simulink model "networkAnalyzer"  (R2023a)
settings: Solver=VariableStepAuto  StartTime=0.0  StopTime=10e-6  RelTol=1e-3
StopFcn:
  | a = smith(SParamObjOut,1,1);
  | a.LineWidth = 3;
  | a.Color = 'red';
undefined symbols (not defined in the file or in its folder): S
libraries: simrfV2elements x4, simrfV2util1 x1, simrfV2testbenches x1
settings Model: Creator=Hossein  LastModifiedBy=Hossein

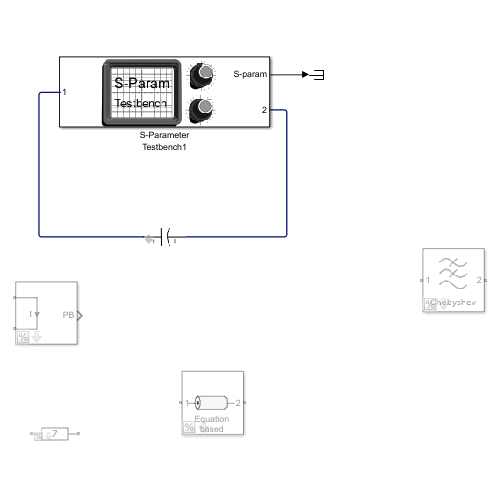
[thumbnail: Simulink's stored preview of the top-level diagram]
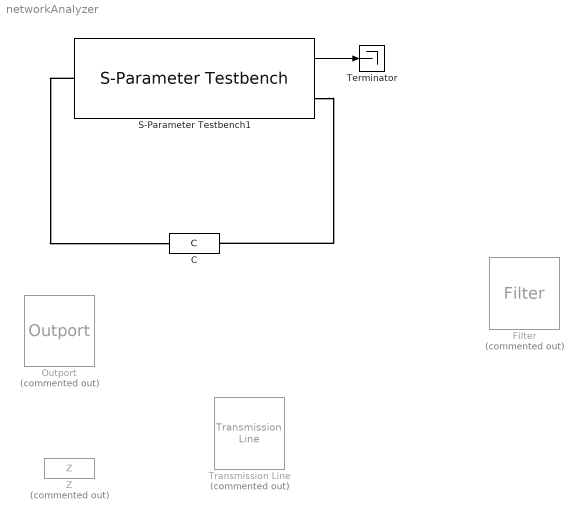
== system networkAnalyzer ==
  C : simrfV2elements/C  classname=capacitor  Capacitance=1e-12 F
  Filter : simrfV2elements/Filter  Commented=on  classname=filter  DesignMethod=Chebyshev  ResponseType=Lowpass  Implementation=LC Tee  ImplementationIdeal=Frequency domain  ImplementationRational=Transfer function  UseFilterOrder=on  FilterOrder=9  PassFreq_lp=1 GHz  PassFreq_hp=2 GHz  PassFreq_bp=[2 3] GHz  PassFreq_bs=[1 4] GHz  PassAtten=10*log10(2)  StopFreq_lp=2 GHz  StopFreq_hp=1 GHz  StopFreq_bp=[1.5 3.5] GHz  StopFreq_bs=[2.1 2.9] GHz  StopAtten=40  Rsrc=50  Rload=50  AutoImpulseLength=off  ImpulseLength=2.5e-10*2048 s  InternalGrounding=on  PlotFuncLeft=Voltage transfer  PlotLeftForm=Magnitude (dB)  PlotRightOnVT=None  PlotRightNoTD=None  PlotRightNoGD=None  PlotRightNoIR=None  PlotRightNoSR=None  PlotRightForm=Imaginary  FreqPoints=[0.75:0.005:1.25]  Freq_unit=GHz  TimePoints=linspace(0,1,1e6+1)  Time_unit=s  XaxisScale=Linear  YaxisScale=Linear  needRedraw=0
  Outport : simrfV2util1/Outport  Commented=on  SensorType=Ideal current  OutputFormat=Real Passband  CarrierFreq=0 Hz  ZL=0  InternalGrounding=off  StepSize=1e-6 s  AutoStep=on  HalfPolyphaseLength=12
  S-Parameter Testbench1 : simrfV2testbenches/S-Parameter Testbench  classname=tbsparam  UseIntConf=on  SimNoise=off  T_amp_dBm=57.0  NumOfPorts=2  MeasureAll=on  SaveS2P=0  ResetableRand=3.8155845709300840e-01  SParamElem=[2 1]  SParamElemPrev=[1 1;2 1;1 2;2 2]  SParamElem1Sel=[1 2;1 2]  SParamElem1SelMapped=[1 2;1 2]  SParamElem1Ind=[1 2 3 4]  SParamElem2Val=[1;2]  InputIdx=1  VarName=SParamObjOut  Fin=2.4e9  Base_bw=800e6  Z0=50  ShowSParam=on  ShowSParamType=Magnitude  MagSparamUnits=Auto  ReImSparamUnits=Auto  InternalGrounding=on  fft_size=1024  Nbins=128  Intermission=3  OS=8  resp=[6.81051648626987e-09;5.8024140195314e-09;3.58265522804047e-09;6.66452894173414e-10;-2.29830488147897e-09;-4.67428137407126e-09;-5.97102098277499e-09;-5.94537038448462e-09;-4.64561861711604e-09;-2.39171175919761e-09;3.02146614802531e-10;2.84404735119469e-09;4.69381960740718e-09;5.47719153734007e-09;5.06068154612974e-09;3.57243094958534e-09;1.366259939602e-09;-1.06150826708262e-09;-3.18309040418601e-09;-4.55343931798306e-09;-4.90300228845816e-09;-4.18984051338105e-09;-2.60123212249622e-09;-5.05981910450121e-10;1.63100066503767e-09;3.35323703526402e-09;4.31630712508652e-09;4.37755410273664e-09;3.67920163757939e-09;2.77705269652491e-09;2.96129531464871e-09;7.1120200677028e-09;2.18299606421558e-08;6.23598544160819e-08;1.63269316723402e-07;4.00396054651843e-07;9.33827347722446e-07;2.08835238509805e-06;4.4976610306672e-06;9.35203499698743e-06;1.8806203403848e-05;3.66229703357968e-05;6.91457717160638e-05;0.000126703493452547;0.000225544772074564;0.000390365110838636;0.000657415791880327;0.00107805759777328;0.00172243928642742;0.00268274593480174;0.00407519716603967;0.00603972153584085;0.00873605359041221;0.0123349736476851;0.0170036224447493;0.0228843469976878;0.0300674092363405;0.0385590946804533;0.0482481936534249;0.0588753004685631;0.07001061092895;0.0810465648285553;0.0912114449704557;0.0996086432816028;0.105283621788724;0.107316735371352;0.104935413468097;0.0976343544391195;0.0852882136126929;0.0682387012558636;0.0473379128100542;0.0239326874790702;-0.000219018604988352;-0.0230997807439736;-0.0426416910645372;-0.056971112585493;-0.0646584952534719;-0.0649370802195157;-0.0578540941489043;-0.0443239056926063;-0.0260644349622775;-0.00541460497265073;0.0149505083913944;0.0323719850072223;0.0445777836518677;0.0500155756815352;0.0480930698267642;0.0392823992156686;0.0250646998199902;0.00771614495830684;-0.0100366513630653;-0.0254404652060814;-0.0361512573431075;-0.040609750820403;-0.0382921967767228;-0.0297911168058924;-0.0167090442506466;-0.00138061048714176;0.0135310307206473;0.0254941930020491;0.0325445139287934;0.0336192652264231;0.0287301008754187;0.0189429989120413;0.00616915572758517;-0.00719464495852944;-0.0187097218303718;-0.026341060203831;-0.0288222277716438;-0.0258723892394917;-0.0182262540822959;-0.00747337715649778;0.00426051684671593;0.0147276156491389;0.0219872110759769;0.0247675993169048;0.0226921959767603;0.016328516091456;0.00705365723689313;-0.00323418431282428;-0.0124989378643042;-0.0189677294627156;-0.0214706685012344;-0.0196536986000975;-0.0140251942169414;-0.00583074630236407;0.00321509414775467;0.0112833612309266;0.016798652509765;0.018746530708132;0.0168601233351881;0.011651374043514;0.00428455388818464;-0.00367838381766407;-0.0106057322490685;-0.0151287962375505;-0.0164117263387738;-0.0143051567759723;-0.00935544535559019;-0.00267156669410891;0.00431917801823937;0.0101734666305566;0.0137285836066262;0.0143325356565713;0.0119621592417434;0.00720806812700198;0.00113337976038217;-0.00496091995827656;-0.00981268853205416;-0.0124588389122865;-0.0124255494971076;-0.0098110335614038;-0.00524684833504798;0.000250580865430648;0.00550399912960573;0.0094259284400338;0.0112427282556662;0.0106461011985825;0.00784256694019479;0.00349366013753298;-0.00143728092288023;-0.00589675524952516;-0.00896497631150719;-0.0100446103639241;-0.00897581265285026;-0.00605566179298668;-0.00196087202808835;0.00240693948276165;0.00611842686995913;0.00841325293231561;0.00885491898650302;0.00741233506927247;0.004453211914578;0.000653443217470372;-0.00315572807088086;-0.00616848715452544;-0.00777405068526528;-0.00767956122390174;-0.0059617359732797;-0.00303858998715499;0.000430238807351771;0.00369116839342279;0.00605951620034682;0.00706248408662136;0.0065325782852347;0.00463321578796572;0.00181324447863779;-0.00129769273768828;-0.0040288277833042;-0.00581216713471303;-0.00629989471799921;-0.00543116121988712;-0.00343567549535713;-0.000775360582626811;0.00196152193691352;0.00418971583470295;0.00545148892238892;0.00550996316427168 ...(+17599 chars)]  respOS=8  AdjustForLargeSig=off  FoutInput=2.4e9  Fout=2400000000  SmallSignalApprox=off  AllSimFreqs=on  SimFreqs=2.1e9
      link override SParam: YLimits=[23.2522,29.4023]  FrequencyVector=[2201562500,2204687500,2207812500,2210937500,2214062500.0000005,2217187500,2220312500,2223437500,2226562500,2229687500.0000005,2232812500,2235937500,2239062500,2242187500,2245312500.0000005,2248437500,2251562500,2254687500,2257812500,2260937500.0000005,2264062500,2267187500,2270312500,2273437500,2276562500.0000005,2279687500,2282812500,2285937500,2289062500,2292187500.0000005,2295312500,2298437500,2301562500,2304687500,2307812500.0000005,2310937500,2314062500,2317187500,2320312500,2323437500.0000005,2326562500,2329687500,2332812500,2335937500,2339062500.0000005,2342187500,2345312500,2348437500,2351562500,2354687500.0000005,2357812500,2360937500,2364062500,2367187500,2370312500.0000005,2373437500,2376562500,2379687500,2382812500,2385937500.0000005,2389062500,2392187500,2395312500,2398437500,2401562500.0000005,2404687500,2407812500,2410937500,2414062500,2417187500.0000005,2420312500,2423437500,2426562500,2429687500,2432812500.0000005,2435937500,2439062500,2442187500,2445312500,2448437500.0000005,2451562500,2454687500,2457812500,2460937500,2464062500.0000005,2467187500,2470312500,2473437500,2476562500,2479687500.0000005,2482812500,2485937500,2489062500,2492187500,2495312500.0000005,2498437500,2501562500.0000005,2504687500,2507812500,2510937500.0000005,2514062500,2517187500.0000005,2520312500,2523437500,2526562500.0000005,2529687500,2532812500.0000005,2535937500,2539062500,2542187500.0000005,2545312500,2548437500.0000005,2551562500,2554687500,2557812500.0000005,2560937500,2564062500.0000005,2567187500,2570312500,2573437500.0000005,2576562500,2579687500.0000005,2582812500,2585937500,2589062500.0000005,2592187500,2595312500.0000005,2598437500]
  Terminator : Terminator
  Transmission Line : simrfV2elements/Transmission Line  Commented=on  classname=xline  Model_type=Equation-based  ConductorBacked=off  StructureMicrostrip=Standard  Parameterization=By characteristic impedance and capacitance  TransDelay=4.7e-9 s  CharImped=25 Ohm  Resistance=0.3 Ohm/m  Inductance=235e-9 H/m  Capacitance=94e-12 F/m  Conductance=5e-6 S/m  LineLength=(3e8/1e9)/4 m  NumSegments=10  InternalGrounding=on  OuterRadius=2.57 mm  InnerRadius=0.725 mm  MuR=1  EpsilonR=2.2  LossTangent=0  SigmaCond=inf S/m  StubMode=Not a stub  Termination=Open  ConductorWidth=0.6 mm  SlotWidth=0.2 mm  Height=0.635 mm  Height_inv=0.635 mm  Height_spd=0.3175 mm  Height_emb=1.37 mm  StripHeight=0.635 mm  Thickness=5 um  SWidth=0.6 mm  Radius=0.67 mm  Separation=1.62 mm  PWidth=5 mm  PSeparation=1 mm  PV=3e8  Loss=0  SourceFreq=User-specified  PlotFreq=[1e9:1e6:3e9] Hz  PlotType=X-Y plane  YParam1=S(1,1)  YFormat1=Magnitude (dB)  YParam2=S(2,2)  YFormat2=Magnitude (dB)  YOption=Linear  XOption=Linear  FitOpt=Share all poles  FitTol=-40  MaxPoles=48  SparamRepresentation=Frequency domain  Freq=1 Ghz  Interp_type=Linear  AutoImpulseLength=off  ImpulseLength=0 s  MagModeling=off
  Z : simrfV2elements/Z  Commented=on  classname=complex_impedance  Impedance_type=Frequency independent  Impedance=25  Freq=1e9 Hz
  wires:
  S-Parameter Testbench1/1 -> Terminator/1
  connections:
  S-Parameter Testbench1/LConn1 -- C/LConn1
  S-Parameter Testbench1/RConn1 -- C/RConn1
